simulink model "EarlyReturn11_2018a"  (R2018a)
settings: Solver=VariableStepAuto  StartTime=0.0  StopTime=0.2  RelTol=1e-3
settings Model: Creator=BEAR  LastModifiedBy=apple

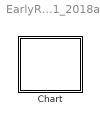
== system EarlyReturn11_2018a ==
  Chart : Stateflow chart  TreatAsAtomicUnit=on

== stateflow chart EarlyReturn11_2018a/Chart ==
  settings: updateMethod=DISCRETE  sampleTime=0.1
  state A
    en: fprintf("en_A")
    ex: fprintf("ex_A")
    state A2
      en: fprintf("en_A2")
      ex: fprintf("ex_A2")
      state A2a
        en: fprintf("en_A2a")
        ex: fprintf("ex_A2a")
    state A3
      en: fprintf("en_A3")
      ex: fprintf("ex_A3")
      state A3a
        en: fprintf("en_A3a")
        ex: fprintf("ex_A3a")
    state A1
      en: fprintf("en_A1")
      ex: fprintf("ex_A1")
    (default) -> A1
    A1 -> A2a
    A2a -> A3a : /{E;fprintf("ta")}
  (default) -> A
  A -> A : E{fprintf("loop")}
  events: E local FUNCTION_CALL_EVENT
